simulink model "Buck_DISM_Matlab_2021a"  (R2021a)
settings: Solver=VariableStepAuto  StartTime=0.0  StopTime=1  RelTol=1e-5
libraries: spsSeriesRLCBranchLib x5, spsCurrentMeasurementLib x3, spsDiodeLib x3, spsDCVoltageSourceLib x1, spsIdealSwitchLib x1, spsTriangleGeneratorLib x1, spsVoltageMeasurementLib x1, spspowerguiLib x1
settings Model: Creator=Asus  LastModifiedBy=Asus
settings DebuggingCC: UnconnectedInputMsg=none  UnconnectedOutputMsg=none  UnconnectedLineMsg=none
settings ModelReferenceCC: EnableRefExpFcnMdlSchedulingChecks=off
settings RTWCC: Description=Generic Real-Time Target  DLArmComputeVersion=20.02.1

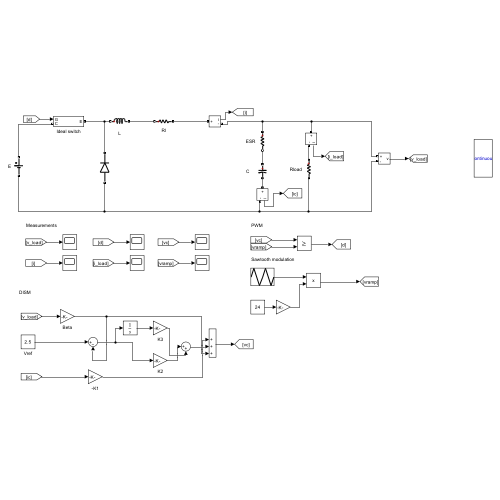
[thumbnail: Simulink's stored preview of the top-level diagram]
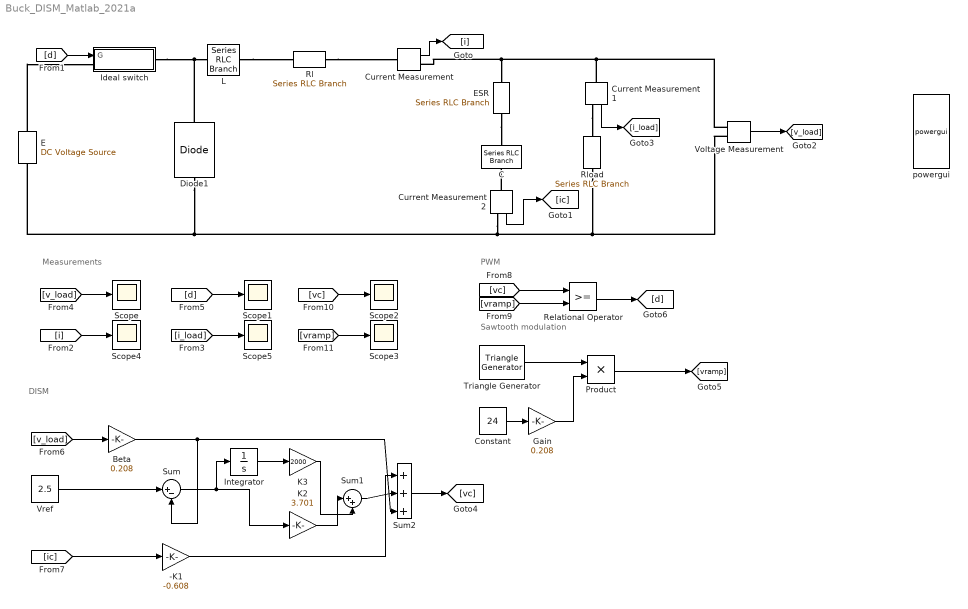
== system Buck_DISM_Matlab_2021a ==
  note: DISM
  note: Sawtooth modulation
  note: Measurements
  note: PWM
  -K1 : Gain  Gain=-0.608
  Beta : Gain  Gain=0.208
  C : spsSeriesRLCBranchLib/Series RLC Branch  LConnTagsString=__new0  RConnTagsString=__new0  BranchType=C  Resistance=1  Inductance=1e-3  SetiL0=off  InitialCurrent=0  Capacitance=0.000150  Setx0=on  InitialVoltage=12  Measurements=None
  Constant : Constant  Value=24
  Current Measurement : spsCurrentMeasurementLib/Current Measurement  PhasorSimulation=off  OutputType=Complex  PSBequivalent=0
  Current Measurement1 : spsCurrentMeasurementLib/Current Measurement  PhasorSimulation=off  OutputType=Complex  PSBequivalent=0
  Current Measurement2 : spsCurrentMeasurementLib/Current Measurement  PhasorSimulation=off  OutputType=Complex  PSBequivalent=0
  Diode1 : spsDiodeLib/Diode  Ron=0.001  Lon=0  Vf=0  IC=0  UseSnubber=0  Rs=inf  Cs=inf  Measurements=off
  E : spsDCVoltageSourceLib/DC Voltage Source  Amplitude=24  Measurements=None
  ESR : spsSeriesRLCBranchLib/Series RLC Branch  LConnTagsString=__new0  RConnTagsString=__new0  BranchType=R  Resistance=0.021  Inductance=1e-3  SetiL0=off  InitialCurrent=0  Capacitance=1e-6  Setx0=off  InitialVoltage=0  Measurements=None
  Gain : Gain  Gain=0.208
  Ideal switch : Subsystem
  Integrator : Integrator
  K2 : Gain  Gain=3.701
  K3 : Gain  Gain=2000
  L : spsSeriesRLCBranchLib/Series RLC Branch  LConnTagsString=__new0  RConnTagsString=__new0  BranchType=L  Resistance=1  Inductance=0.040  SetiL0=off  InitialCurrent=0  Capacitance=1e-6  Setx0=off  InitialVoltage=0  Measurements=None
  Product : Product
  Relational Operator : RelationalOperator  OutDataTypeStr=boolean  RndMeth=Simplest
  Rl : spsSeriesRLCBranchLib/Series RLC Branch  LConnTagsString=__new0  RConnTagsString=__new0  BranchType=R  Resistance=0.12  Inductance=1e-3  SetiL0=off  InitialCurrent=0  Capacitance=1e-6  Setx0=off  InitialVoltage=0  Measurements=None
  Rload : spsSeriesRLCBranchLib/Series RLC Branch  LConnTagsString=__new0  RConnTagsString=__new0  BranchType=R  Resistance=3  Inductance=1e-3  SetiL0=off  InitialCurrent=0  Capacitance=1e-6  Setx0=off  InitialVoltage=0  Measurements=None
  Scope{,1..5} (6 alike) : Scope
  Sum : Sum  Inputs=|+-
  Sum1 : Sum  Inputs=|++
  Sum2 : Sum  Inputs=|+++
  Triangle Generator : spsTriangleGeneratorLib/Triangle Generator  Freq=20000  Phase=90  Ts=0
  Voltage Measurement : spsVoltageMeasurementLib/Voltage Measurement  PhasorSimulation=off  OutputType=Complex  PSBequivalent=0
  Vref : Constant  Value=2.5
  powergui : spspowerguiLib/powergui  Priority=1  SimulationMode=Continuous  SampleTime=1/20000000  frequency=60  Iterations=50  frequencyindice=0  Pbase=100e6  ErrMax=1e-4  UnitsV=kV  UnitsW=MW  buscounter=0  FunctionMessages=off  echomessages=off  EnableUseOfTLC=off  CurrentSourceSwitches=off  DisableSnubberDevices=off  DisableRonSwitches=off  DisableVfSwitches=off  DisplayEquations=off  AutomaticDiscreteSolvers=off  SolverType=Tustin/Backward Euler (TBE)  Interpol=off  ExternalGateDelay=off  methode=off  Ts=100  x0status=blocks  SPID=on  SwTol=0  HookPort=off  NonlinearTolerance=1e-4  nMaxIteration=100  ContinueOnMaxIteration=off  RestoreLinks=warning  ResistiveCurrentMeasurement=off  Frange=[0:2:500]  Ylog=off  Xlog=on  ShowGrid=off  save=off  variable=ZData  structure=0  ZoomFFT=off  StartTime=0.0  cycles=1  DisplayStyle=1  fundamental=60  FreqAxis=off  MaxFrequency=1000  frequencyindicesteady=1  RmsSteady=1  display=off
  wires:
  [v_load] -> Scope/1
  Current Measurement/1 -> [i]
  Voltage Measurement/1 -> [v_load]
  [i_load] -> Scope5/1
  [i] -> Scope4/1
  [d] -> Ideal switch/1(G)
  Current Measurement1/1 -> [i_load]
  [d] -> Scope1/1
  [v_load] -> Beta/1
  Beta/1 -> Sum2/3, Sum/2
  Vref/1 -> Sum/1
  Sum/1 -> Integrator/1, K2/1
  Integrator/1 -> K3/1
  K2/1 -> Sum1/1
  Sum1/1 -> Sum2/2
  Current Measurement2/1 -> [ic]
  [ic] -> -K1/1
  -K1/1 -> Sum2/1
  Sum2/1 -> [vc]
  Gain/1 -> Product/2
  Constant/1 -> Gain/1
  Product/1 -> [vramp]
  [vc] -> Relational Operator/1
  [vramp] -> Relational Operator/2
  Relational Operator/1 -> [d]
  [vramp] -> Scope3/1
  [vc] -> Scope2/1
  K3/1 -> Sum1/2
  Triangle Generator/1 -> Product/1
  connections:
  Voltage Measurement/LConn1 -- ESR/LConn1 -- Current Measurement/RConn1 -- Current Measurement1/LConn1
  E/LConn1 -- Current Measurement2/RConn1 -- Rload/RConn1 -- Voltage Measurement/LConn2 -- Diode1/LConn1
  L/LConn1 -- Ideal switch/RConn1 -- Diode1/RConn1
  L/RConn1 -- Rl/LConn1
  E/RConn1 -- Ideal switch/LConn1
  Current Measurement1/RConn1 -- Rload/LConn1
  Rl/RConn1 -- Current Measurement/LConn1
  ESR/RConn1 -- C/LConn1
  Current Measurement2/LConn1 -- C/RConn1

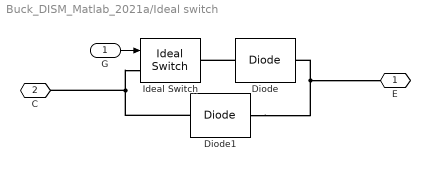
== system Buck_DISM_Matlab_2021a/Ideal switch ==
  G : Inport
  Diode : spsDiodeLib/Diode  Ron=0  Lon=0  Vf=0  IC=0  UseSnubber=0  Rs=inf  Cs=inf  Measurements=off
  Diode1 : spsDiodeLib/Diode  Ron=0  Lon=0  Vf=0  IC=0  UseSnubber=0  Rs=inf  Cs=inf  Measurements=off
  Ideal Switch : spsIdealSwitchLib/Ideal Switch  Ron=0  Lon=0  IC=1  Rs=inf  Cs=inf  Measurements=off
  E : PMIOPort  Side=Right
  C : PMIOPort  Port=2  Side=Left
  wires:
  G/1 -> Ideal Switch/1
  connections:
  Diode/LConn1 -- Ideal Switch/RConn1
  Diode1/RConn1 -- Ideal Switch/LConn1 -- C/RConn1
  Diode1/LConn1 -- E/RConn1 -- Diode/RConn1
